simulink model "IEEE_39_IBR_Simplified"  (R2023b)
settings: Solver=FixedStepAuto  StartTime=0  StopTime=20  FixedStep=Ts  MaxStep=1/60  RelTol=1e-3  AbsTol=1e-2  EnableMultiTasking=on
PreLoadFcn:
  | NE39bus_data;
  | PSSMODEL=1;
  | LPSS=0;
  | WAPSS=0;
  | WAPSS2=0;
values from neighbouring files (symbols this model uses):
  Dt = 0    [SG_para.m]
  dw0_sm = 0    [SG_para.m]
  Emax = 1    [SG_para.m]
  Emin = 0.5    [SG_para.m]
  Fg = [0.1,0.1,0.1]    [SG_para.m]
  fn_sm = 60*ones(1,10)    [SG_para.m]
  H_sm = [5,3.03,3.58,2.86,2.6,3.48,2.64,2.43,3.45,4.2]*10    [SG_para.m]
  ia0_sm = 0.75*0    (= 0)    [SG_para.m]
  ib0_sm = 0.75*0    (= 0)    [SG_para.m]
  ic0_sm = 0.75*0    (= 0)    [SG_para.m]
  Kd_sm = 6*ones(1,10)    [SG_para.m]
  Ke = 200    [SG_para.m]
  Kg = [0.95,0.95,0.95]    [SG_para.m]
  Ks = 2    [SG_para.m]
  line = [     1	2	0.0035	0.0411	0.6987	0	100	345 ... (first row only)    [SG_para.m]
  p = 1    [SG_para.m]
  pha0_sm = -24.95*0    (= 0)    [SG_para.m]
  phb0_sm = -144.94*0    (= 0)    [SG_para.m]
  phc0_sm = 95.05*0    (= 0)    [SG_para.m]
  Pn_sm = [1000,1000,1000,1000,1000,1000,1000,1000,1000,1000]    [SG_para.m]
  Pref_sm = [1000 520.81 650 632 508 650 560 540 830 250]./Pn_sm    [SG_para.m]
  R = 1e-3    (= 0.001)    [SG_para.m]
  Rg = [0.05,0.05,0.05]    [SG_para.m]
  rs = 2.8544e-3    (= 0.0028544)    [SG_para.m]
  s = 1    [SG_para.m]
  s1 = 10    [SG_para.m]
  T1 = 0.05    [SG_para.m]
  T2 = 0.5    [SG_para.m]
  T3 = 0.5    [SG_para.m]
  Te = 0.05    [SG_para.m]
  Tfa = 3    [SG_para.m]
  Tfb = 10    [SG_para.m]
  Tg = [10,10,10]    [SG_para.m]
  theta0_sm = -94.3*0    (= 0)    [SG_para.m]
  Ts = 5e-5    (= 5e-05)    [SG_para.m]
  Ts1 = 0.18    [SG_para.m]
  Ts2 = 2    [SG_para.m]
  Ts3 = 5    [SG_para.m]
  Ts4 = 10    [SG_para.m]
  Ts5 = 15    [SG_para.m]
  Un_sm = [345,22,22,22,22,22,22,22,345,22]    [SG_para.m]
  Vmax = inf    [SG_para.m]
  Vmin = 0    [SG_para.m]
  Vref_sm = 1*ones(1,10)    [SG_para.m]
  xd = xd_t    (= 0.296)    [SG_para.m]
undefined symbols (not defined in the file or in its folder): D1, D11, Delta, Ka, Kf, Ta, Tf
libraries: spsThreePhaseVIMeasurementLib x41, spsThreePhaseFaultLib x39, spsThreePhaseSeriesRLCBranchLib x36, spsThreePhaseParallelRLCLoadLib x20, spsThreePhaseTransformerTwoWindingsLib x13, spsSimplifiedSynchronousMachinepuUnitsLib x10, spsLoadFlowBusLib x10, Inverter_based_Resources_IBRs x10, spsThreePhaseBreakerLib x2, spsSequenceAnalyzerLib x2, spsMultimeterLib x1, eePowerMeasurement x1
(part 5 of 5)

== system IEEE_39_IBR_Simplified/A3/G6/Controllers/Governor IEEE TGOV1 ==
  dw : Inport
  Pref : Inport  Port=2
  Gain : Gain  Gain=1/R
  Gain1 : Gain  Gain=Dt
  Saturation : Saturate  UpperLimit=Vmax  LowerLimit=Vmin
  Scope : Scope  NumInputPorts=3
  Scope1 : Scope
  Sum : Sum  Inputs=|+-
  Sum1 : Sum  Inputs=|+-
  Transfer Fcn : TransferFcn  Denominator=[T1 1]
  Transfer Fcn1 : TransferFcn  Numerator=[T2 1]  Denominator=[T3 1]
  Transfer Fcn2 : TransferFcn  Numerator=[1 1]  Denominator=[10 1]
  Pm : Outport  VectorParamsAs1DForOutWhenUnconnected=off
  wires:
  Transfer Fcn/1 -> Scope1/1, Saturation/1
  Sum1/1 -> Scope/2, Transfer Fcn/1
  Gain1/1 -> Sum/2
  Saturation/1 -> Transfer Fcn1/1
  Sum/1 -> Pm/1
  dw/1 -> Transfer Fcn2/1
  Transfer Fcn1/1 -> Scope/3, Sum/1
  Gain/1 -> Sum1/2
  Pref/1 -> Scope/1, Sum1/1
  Transfer Fcn2/1 -> Gain1/1, Gain/1

== system IEEE_39_IBR_Simplified/A3/G6/Controllers/PSS IEEE PSS1A ==
  dP : Inport
  Gain : Gain  Gain=Ks
  Transfer Fcn : TransferFcn  Numerator=[Ts1 1]  Denominator=[Ts2 1]
  Transfer Fcn1 : TransferFcn  Numerator=[Ts5 0]  Denominator=[Ts5 1]
  Transfer Fcn2 : TransferFcn  Numerator=[Ts3 1]  Denominator=[Ts4 1]
  Vs : Outport  VectorParamsAs1DForOutWhenUnconnected=off
  wires:
  Transfer Fcn/1 -> Transfer Fcn2/1
  Gain/1 -> Transfer Fcn1/1
  dP/1 -> Transfer Fcn/1
  Transfer Fcn2/1 -> Gain/1
  Transfer Fcn1/1 -> Vs/1

== system IEEE_39_IBR_Simplified/A3/G7/Controllers/AVR IEEE SEXS\ST1A ==
  Vc : Inport
  Vs : Inport  Port=2
  Vref : Inport  Port=3
  AVR IEEE ST1a : Subsystem  Commented=on
  AVR SEXS : Subsystem
  Sum1 : Sum  Inputs=+-+
  Ef : Outport  VectorParamsAs1DForOutWhenUnconnected=off
  wires:
  Vc/1 -> Sum1/2
  Vref/1 -> Sum1/1
  Vs/1 -> Sum1/3
  Sum1/1 -> AVR SEXS/1(dV)
  AVR SEXS/1(Ef) -> Ef/1

== system IEEE_39_IBR_Simplified/A3/G7/Controllers/Governor Simplified ==
  dw : Inport
  Pref : Inport  Port=2
  Gain : Gain  Gain=Kg(1)/Rg(1)
  Saturation : Saturate  UpperLimit=Vmax  LowerLimit=Vmin
  Sum1 : Sum  Inputs=|+-
  Transfer Fcn : TransferFcn  Numerator=[Fg(1)*Tg(1) 1]  Denominator=[Tg(1) 1]
  Pm : Outport  VectorParamsAs1DForOutWhenUnconnected=off
  wires:
  Transfer Fcn/1 -> Gain/1
  dw/1 -> Transfer Fcn/1
  Pref/1 -> Sum1/1
  Sum1/1 -> Saturation/1
  Gain/1 -> Sum1/2
  Saturation/1 -> Pm/1

== system IEEE_39_IBR_Simplified/A3/G7/Controllers/Governor IEEE TGOV1 ==
  dw : Inport
  Pref : Inport  Port=2
  Gain : Gain  Gain=1/R
  Gain1 : Gain  Gain=Dt
  Saturation : Saturate  UpperLimit=inf  LowerLimit=Vmin
  Scope : Scope  NumInputPorts=3
  Scope1 : Scope
  Sum : Sum  Inputs=|+-
  Sum1 : Sum  Inputs=|+-
  Transfer Fcn : TransferFcn  Denominator=[T1 1]
  Transfer Fcn1 : TransferFcn  Numerator=[T2 1]  Denominator=[T3 1]
  Transfer Fcn2 : TransferFcn  Numerator=[1 1]  Denominator=[10 1]
  Pm : Outport  VectorParamsAs1DForOutWhenUnconnected=off
  wires:
  Transfer Fcn/1 -> Scope1/1, Saturation/1
  Sum1/1 -> Scope/2, Transfer Fcn/1
  Gain1/1 -> Sum/2
  Saturation/1 -> Transfer Fcn1/1
  Sum/1 -> Pm/1
  dw/1 -> Transfer Fcn2/1
  Transfer Fcn1/1 -> Scope/3, Sum/1
  Gain/1 -> Sum1/2
  Pref/1 -> Scope/1, Sum1/1
  Transfer Fcn2/1 -> Gain1/1, Gain/1

== system IEEE_39_IBR_Simplified/A3/G7/Controllers/PSS IEEE PSS1A ==
  dP : Inport
  Gain : Gain  Gain=Ks
  Transfer Fcn : TransferFcn  Numerator=[Ts1 1]  Denominator=[Ts2 1]
  Transfer Fcn1 : TransferFcn  Numerator=[Ts5 0]  Denominator=[Ts5 1]
  Transfer Fcn2 : TransferFcn  Numerator=[Ts3 1]  Denominator=[Ts4 1]
  Vs : Outport  VectorParamsAs1DForOutWhenUnconnected=off
  wires:
  Transfer Fcn/1 -> Transfer Fcn2/1
  Gain/1 -> Transfer Fcn1/1
  dP/1 -> Transfer Fcn/1
  Transfer Fcn2/1 -> Gain/1
  Transfer Fcn1/1 -> Vs/1

== system IEEE_39_IBR_Simplified/A1/G10/Controllers/AVR IEEE SEXS\ST1A/AVR IEEE ST1a ==
  dV : Inport
  Sum : Sum  Inputs=|+-
  Transfer Fcn1 : TransferFcn  Numerator=[Ka]  Denominator=[Ta 1]
  Transfer Fcn2 : TransferFcn  Numerator=[Kf 0]  Denominator=[Tf 1]
  Ef : Outport  VectorParamsAs1DForOutWhenUnconnected=off
  wires:
  Transfer Fcn1/1 -> Transfer Fcn2/1, Ef/1
  Sum/1 -> Transfer Fcn1/1
  dV/1 -> Sum/1
  Transfer Fcn2/1 -> Sum/2

== system IEEE_39_IBR_Simplified/A1/G10/Controllers/AVR IEEE SEXS\ST1A/AVR SEXS ==
  dV : Inport
  Saturation : Saturate  UpperLimit=Emax  LowerLimit=Emin
  Transfer Fcn : TransferFcn  Numerator=[Tfa 1]  Denominator=[Tfb 1]
  Transfer Fcn1 : TransferFcn  Numerator=[Ke]  Denominator=[Te 1]
  Ef : Outport  VectorParamsAs1DForOutWhenUnconnected=off
  wires:
  Saturation/1 -> Ef/1
  Transfer Fcn1/1 -> Saturation/1
  Transfer Fcn/1 -> Transfer Fcn1/1
  dV/1 -> Transfer Fcn/1

== system IEEE_39_IBR_Simplified/A1/G8/Controllers/AVR IEEE SEXS\ST1A/AVR IEEE ST1a ==
  dV : Inport
  Sum : Sum  Inputs=|+-
  Transfer Fcn1 : TransferFcn  Numerator=[Ka]  Denominator=[Ta 1]
  Transfer Fcn2 : TransferFcn  Numerator=[Kf 0]  Denominator=[Tf 1]
  Ef : Outport  VectorParamsAs1DForOutWhenUnconnected=off
  wires:
  Transfer Fcn1/1 -> Transfer Fcn2/1, Ef/1
  Sum/1 -> Transfer Fcn1/1
  dV/1 -> Sum/1
  Transfer Fcn2/1 -> Sum/2

== system IEEE_39_IBR_Simplified/A1/G8/Controllers/AVR IEEE SEXS\ST1A/AVR SEXS ==
  dV : Inport
  Saturation : Saturate  UpperLimit=Emax  LowerLimit=Emin
  Transfer Fcn : TransferFcn  Numerator=[Tfa 1]  Denominator=[Tfb 1]
  Transfer Fcn1 : TransferFcn  Numerator=[Ke]  Denominator=[Te 1]
  Ef : Outport  VectorParamsAs1DForOutWhenUnconnected=off
  wires:
  Saturation/1 -> Ef/1
  Transfer Fcn1/1 -> Saturation/1
  Transfer Fcn/1 -> Transfer Fcn1/1
  dV/1 -> Transfer Fcn/1

== system IEEE_39_IBR_Simplified/A1/G9/Controllers/AVR IEEE SEXS\ST1A/AVR IEEE ST1a ==
  dV : Inport
  Sum : Sum  Inputs=|+-
  Transfer Fcn1 : TransferFcn  Numerator=[Ka]  Denominator=[Ta 1]
  Transfer Fcn2 : TransferFcn  Numerator=[Kf 0]  Denominator=[Tf 1]
  Ef : Outport  VectorParamsAs1DForOutWhenUnconnected=off
  wires:
  Transfer Fcn1/1 -> Transfer Fcn2/1, Ef/1
  Sum/1 -> Transfer Fcn1/1
  dV/1 -> Sum/1
  Transfer Fcn2/1 -> Sum/2

== system IEEE_39_IBR_Simplified/A1/G9/Controllers/AVR IEEE SEXS\ST1A/AVR SEXS ==
  dV : Inport
  Saturation : Saturate  UpperLimit=Emax  LowerLimit=Emin
  Transfer Fcn : TransferFcn  Numerator=[Tfa 1]  Denominator=[Tfb 1]
  Transfer Fcn1 : TransferFcn  Numerator=[Ke]  Denominator=[Te 1]
  Ef : Outport  VectorParamsAs1DForOutWhenUnconnected=off
  wires:
  Saturation/1 -> Ef/1
  Transfer Fcn1/1 -> Saturation/1
  Transfer Fcn/1 -> Transfer Fcn1/1
  dV/1 -> Transfer Fcn/1

== system IEEE_39_IBR_Simplified/A2/G1/Controllers/AVR IEEE SEXS\ST1A/AVR IEEE ST1a ==
  dV : Inport
  Sum : Sum  Inputs=|+-
  Transfer Fcn1 : TransferFcn  Numerator=[Ka]  Denominator=[Ta 1]
  Transfer Fcn2 : TransferFcn  Numerator=[Kf 0]  Denominator=[Tf 1]
  Ef : Outport  VectorParamsAs1DForOutWhenUnconnected=off
  wires:
  Transfer Fcn1/1 -> Transfer Fcn2/1, Ef/1
  Sum/1 -> Transfer Fcn1/1
  dV/1 -> Sum/1
  Transfer Fcn2/1 -> Sum/2

== system IEEE_39_IBR_Simplified/A2/G1/Controllers/AVR IEEE SEXS\ST1A/AVR SEXS ==
  dV : Inport
  Saturation : Saturate  UpperLimit=Emax  LowerLimit=Emin
  Transfer Fcn : TransferFcn  Numerator=[Tfa 1]  Denominator=[Tfb 1]
  Transfer Fcn1 : TransferFcn  Numerator=[Ke]  Denominator=[Te 1]
  Ef : Outport  VectorParamsAs1DForOutWhenUnconnected=off
  wires:
  Saturation/1 -> Ef/1
  Transfer Fcn1/1 -> Saturation/1
  Transfer Fcn/1 -> Transfer Fcn1/1
  dV/1 -> Transfer Fcn/1

== system IEEE_39_IBR_Simplified/A2/G2/Controllers/AVR IEEE SEXS\ST1A/AVR IEEE ST1a ==
  dV : Inport
  Sum : Sum  Inputs=|+-
  Transfer Fcn1 : TransferFcn  Numerator=[Ka]  Denominator=[Ta 1]
  Transfer Fcn2 : TransferFcn  Numerator=[Kf 0]  Denominator=[Tf 1]
  Ef : Outport  VectorParamsAs1DForOutWhenUnconnected=off
  wires:
  Transfer Fcn1/1 -> Transfer Fcn2/1, Ef/1
  Sum/1 -> Transfer Fcn1/1
  dV/1 -> Sum/1
  Transfer Fcn2/1 -> Sum/2

== system IEEE_39_IBR_Simplified/A2/G2/Controllers/AVR IEEE SEXS\ST1A/AVR SEXS ==
  dV : Inport
  Saturation : Saturate  UpperLimit=Emax  LowerLimit=Emin
  Transfer Fcn : TransferFcn  Numerator=[Tfa 1]  Denominator=[Tfb 1]
  Transfer Fcn1 : TransferFcn  Numerator=[Ke]  Denominator=[Te 1]
  Ef : Outport  VectorParamsAs1DForOutWhenUnconnected=off
  wires:
  Saturation/1 -> Ef/1
  Transfer Fcn1/1 -> Saturation/1
  Transfer Fcn/1 -> Transfer Fcn1/1
  dV/1 -> Transfer Fcn/1

== system IEEE_39_IBR_Simplified/A2/G3/Controllers/AVR IEEE SEXS\ST1A/AVR IEEE ST1a ==
  dV : Inport
  Sum : Sum  Inputs=|+-
  Transfer Fcn1 : TransferFcn  Numerator=[Ka]  Denominator=[Ta 1]
  Transfer Fcn2 : TransferFcn  Numerator=[Kf 0]  Denominator=[Tf 1]
  Ef : Outport  VectorParamsAs1DForOutWhenUnconnected=off
  wires:
  Transfer Fcn1/1 -> Transfer Fcn2/1, Ef/1
  Sum/1 -> Transfer Fcn1/1
  dV/1 -> Sum/1
  Transfer Fcn2/1 -> Sum/2

== system IEEE_39_IBR_Simplified/A2/G3/Controllers/AVR IEEE SEXS\ST1A/AVR SEXS ==
  dV : Inport
  Saturation : Saturate  UpperLimit=Emax  LowerLimit=Emin
  Scope : Scope  NumInputPorts=3
  Transfer Fcn : TransferFcn  Numerator=[Tfa 1]  Denominator=[Tfb 1]
  Transfer Fcn1 : TransferFcn  Numerator=[Ke]  Denominator=[Te 1]
  Ef : Outport  VectorParamsAs1DForOutWhenUnconnected=off
  wires:
  Saturation/1 -> Scope/3, Ef/1
  Transfer Fcn1/1 -> Scope/2, Saturation/1
  Transfer Fcn/1 -> Transfer Fcn1/1
  dV/1 -> Scope/1, Transfer Fcn/1

== system IEEE_39_IBR_Simplified/A3/G4/Controllers/AVR IEEE SEXS\ST1A/AVR IEEE ST1a ==
  dV : Inport
  Sum : Sum  Inputs=|+-
  Transfer Fcn1 : TransferFcn  Numerator=[Ka]  Denominator=[Ta 1]
  Transfer Fcn2 : TransferFcn  Numerator=[Kf 0]  Denominator=[Tf 1]
  Ef : Outport  VectorParamsAs1DForOutWhenUnconnected=off
  wires:
  Transfer Fcn1/1 -> Transfer Fcn2/1, Ef/1
  Sum/1 -> Transfer Fcn1/1
  dV/1 -> Sum/1
  Transfer Fcn2/1 -> Sum/2

== system IEEE_39_IBR_Simplified/A3/G4/Controllers/AVR IEEE SEXS\ST1A/AVR SEXS ==
  dV : Inport
  Saturation : Saturate  UpperLimit=Emax  LowerLimit=Emin
  Transfer Fcn : TransferFcn  Numerator=[Tfa 1]  Denominator=[Tfb 1]
  Transfer Fcn1 : TransferFcn  Numerator=[Ke]  Denominator=[Te 1]
  Ef : Outport  VectorParamsAs1DForOutWhenUnconnected=off
  wires:
  Saturation/1 -> Ef/1
  Transfer Fcn1/1 -> Saturation/1
  Transfer Fcn/1 -> Transfer Fcn1/1
  dV/1 -> Transfer Fcn/1

== system IEEE_39_IBR_Simplified/A3/G5/Controllers/AVR IEEE SEXS\ST1A/AVR IEEE ST1a ==
  dV : Inport
  Sum : Sum  Inputs=|+-
  Transfer Fcn1 : TransferFcn  Numerator=[Ka]  Denominator=[Ta 1]
  Transfer Fcn2 : TransferFcn  Numerator=[Kf 0]  Denominator=[Tf 1]
  Ef : Outport  VectorParamsAs1DForOutWhenUnconnected=off
  wires:
  Transfer Fcn1/1 -> Transfer Fcn2/1, Ef/1
  Sum/1 -> Transfer Fcn1/1
  dV/1 -> Sum/1
  Transfer Fcn2/1 -> Sum/2

== system IEEE_39_IBR_Simplified/A3/G5/Controllers/AVR IEEE SEXS\ST1A/AVR SEXS ==
  dV : Inport
  Saturation : Saturate  UpperLimit=Emax  LowerLimit=Emin
  Transfer Fcn : TransferFcn  Numerator=[Tfa 1]  Denominator=[Tfb 1]
  Transfer Fcn1 : TransferFcn  Numerator=[Ke]  Denominator=[Te 1]
  Ef : Outport  VectorParamsAs1DForOutWhenUnconnected=off
  wires:
  Saturation/1 -> Ef/1
  Transfer Fcn1/1 -> Saturation/1
  Transfer Fcn/1 -> Transfer Fcn1/1
  dV/1 -> Transfer Fcn/1

== system IEEE_39_IBR_Simplified/A3/G6/Controllers/AVR IEEE SEXS\ST1A/AVR IEEE ST1a ==
  dV : Inport
  Sum : Sum  Inputs=|+-
  Transfer Fcn1 : TransferFcn  Numerator=[Ka]  Denominator=[Ta 1]
  Transfer Fcn2 : TransferFcn  Numerator=[Kf 0]  Denominator=[Tf 1]
  Ef : Outport  VectorParamsAs1DForOutWhenUnconnected=off
  wires:
  Transfer Fcn1/1 -> Transfer Fcn2/1, Ef/1
  Sum/1 -> Transfer Fcn1/1
  dV/1 -> Sum/1
  Transfer Fcn2/1 -> Sum/2

== system IEEE_39_IBR_Simplified/A3/G6/Controllers/AVR IEEE SEXS\ST1A/AVR SEXS ==
  dV : Inport
  Saturation : Saturate  UpperLimit=Emax  LowerLimit=Emin
  Transfer Fcn : TransferFcn  Numerator=[Tfa 1]  Denominator=[Tfb 1]
  Transfer Fcn1 : TransferFcn  Numerator=[Ke]  Denominator=[Te 1]
  Ef : Outport  VectorParamsAs1DForOutWhenUnconnected=off
  wires:
  Saturation/1 -> Ef/1
  Transfer Fcn1/1 -> Saturation/1
  Transfer Fcn/1 -> Transfer Fcn1/1
  dV/1 -> Transfer Fcn/1

== system IEEE_39_IBR_Simplified/A3/G7/Controllers/AVR IEEE SEXS\ST1A/AVR IEEE ST1a ==
  dV : Inport
  Sum : Sum  Inputs=|+-
  Transfer Fcn1 : TransferFcn  Numerator=[Ka]  Denominator=[Ta 1]
  Transfer Fcn2 : TransferFcn  Numerator=[Kf 0]  Denominator=[Tf 1]
  Ef : Outport  VectorParamsAs1DForOutWhenUnconnected=off
  wires:
  Transfer Fcn1/1 -> Transfer Fcn2/1, Ef/1
  Sum/1 -> Transfer Fcn1/1
  dV/1 -> Sum/1
  Transfer Fcn2/1 -> Sum/2

== system IEEE_39_IBR_Simplified/A3/G7/Controllers/AVR IEEE SEXS\ST1A/AVR SEXS ==
  dV : Inport
  Saturation : Saturate  UpperLimit=Emax  LowerLimit=Emin
  Transfer Fcn : TransferFcn  Numerator=[Tfa 1]  Denominator=[Tfb 1]
  Transfer Fcn1 : TransferFcn  Numerator=[Ke]  Denominator=[Te 1]
  Ef : Outport  VectorParamsAs1DForOutWhenUnconnected=off
  wires:
  Saturation/1 -> Ef/1
  Transfer Fcn1/1 -> Saturation/1
  Transfer Fcn/1 -> Transfer Fcn1/1
  dV/1 -> Transfer Fcn/1
